simulink model "MMC_SwitchingModel_20250511"  (R2024b)
settings: Solver=VariableStepAuto  StartTime=0.0  StopTime=0.35  RelTol=1e-3
values from neighbouring files (symbols this model uses):
  Ceq = 3e-3    (= 0.003)    [param_allsim_20250429.m]
  f0 = 50    [param_allsim_20250429.m]
  Fc = 1e3    (= 1000)    [param_allsim_20250429.m]
  L_ac = 100e-6    (= 0.0001)    [param_allsim_20250429.m]
  L_arm = 1e-3    (= 0.001)    [param_allsim_20250429.m]
  m_Delta_0 = m_Delta_0_n    (= 0)    [param_allsim_20250429.m]
  m_Delta_d = M_Delta*sin(Phi_Delta)    [param_allsim_20250429.m]
  m_Delta_q = -M_Delta*cos(Phi_Delta)    [param_allsim_20250429.m]
  m_Sigma_0 = m_Sigma_0_n    (= 1)    [param_allsim_20250429.m]
  m_Sigma_d = M_Sigma*sin(Phi_Sigma)    [param_allsim_20250429.m]
  m_Sigma_q = -M_Sigma*cos(Phi_Sigma)    [param_allsim_20250429.m]
  N = 6    [param_allsim_20250429.m]
  R_ac = 1    [param_allsim_20250429.m]
  R_arm = 1e-2    (= 0.01)    [param_allsim_20250429.m]
  VDC = 800    [param_allsim_20250429.m]
undefined symbols (not defined in the file or in its folder): C_SM
libraries: spsVoltageMeasurementLib x11, spsCurrentMeasurementLib x8, spsSeriesRLCBranchLib x6, spsHalfBridgeMMCLib x6, spsPWMGeneratorMultilevelLib x6, spsabctodq0Lib x6, spsDCVoltageSourceLib x2, spsdq0toabcLib x2, spsGroundLib x1, spsThreePhaseSeriesRLCBranchLib x1, spsMeanLib x1, spspowerguiLib x1
(part 1 of 2)
settings Model: Creator=ana  LastModifiedBy=ana

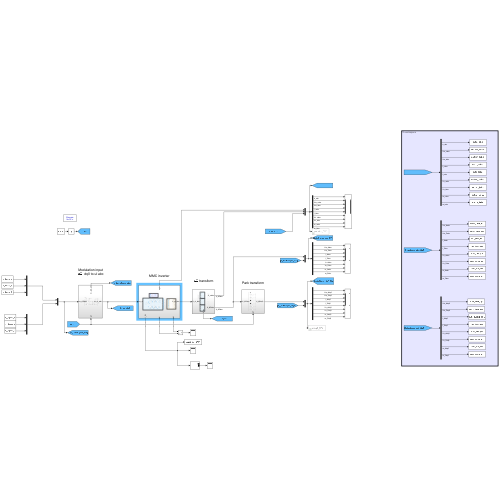
[thumbnail: Simulink's stored preview of the top-level diagram]
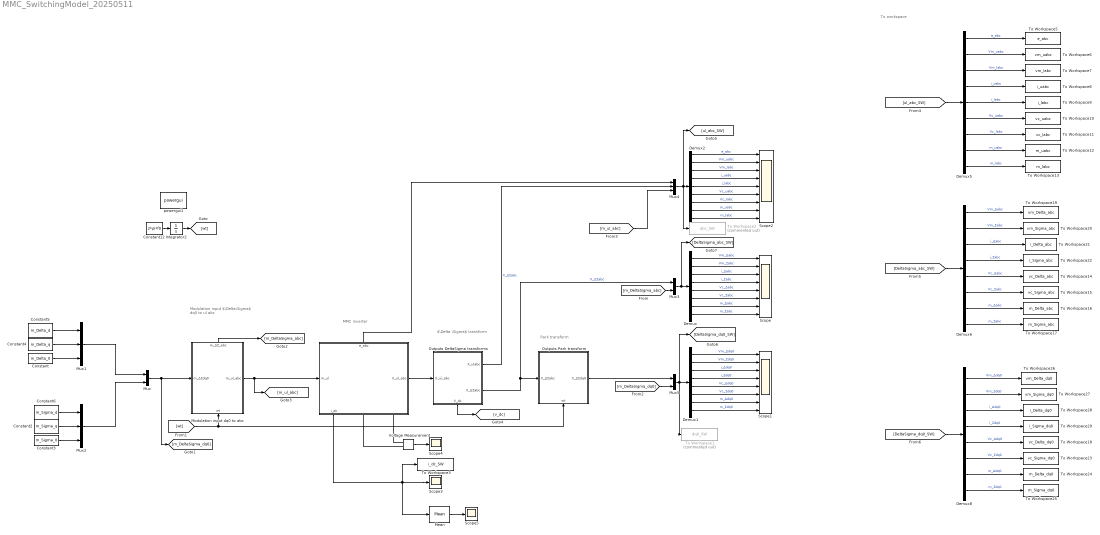
== system MMC_SwitchingModel_20250511 ==
  note: Modulation input
      | $\Delta\Sigma$ dq0 to ul abc
  note: MMC inverter
  note: $\Delta \Sigma$ transform
  note: Park transform
  note: To workspace
  " " : Subsystem
      settings: PortSchema="{\"entries\":[{\"content\":{\"sides\":[{\"content\":{\"connectorIds\":[\"In1\"]},\"type\":\"ConnectorPlacement.EquallySpacedRectSide\",\"uuid\":\"1684c177-0f69-459b-8ce9-190a6cc7c2f7\"},{\"content\":{\"connectorIds\":[\"Out1\"],\"side\":\"RIGHT\"},\"type\":\"ConnectorPlacement.EquallySpacedRectSide\",\"uuid\":\"0bff5431-30f2-45f3-9612-3e8ee114177b\"},{\"content\":{\"connectorIds\":[\"Out3\"],\"side\":\"TOP\"},\"type\":\"ConnectorPlacement.EquallySpacedRectSide\",\"uuid\":\"5880dbee-f5bf-4d11-b41f-6e883d19a036\"},{\"content\":{\"connectorIds\":[\"Out2\",\"RConn1\",\"RConn2\"],\"side\":\"BOTTOM\"},\"type\":\"ConnectorPlacement.EquallySpacedRectSide\",\"uuid\":\"e7f28e42-6c15-4753-aad9-7fd8153dbb2b\"}]},\"type\":\"ConnectorPlacement.EquallySpacedConnector\",\"uuid\":\"d5dc9c97-4c49-4fa9-8e0e-631ade92c721\"}],\"packageUris\":[\"http://schema.mathworks.com/mf0/Connector/R2020b\"],\"version\":\"1.0\"}"
  Constant : Constant  Value=m_Delta_0
  Constant12 : Constant  Value=2*pi*f0
  Constant2 : Constant  Value=m_Sigma_q
  Constant3 : Constant  Value=m_Sigma_0
  Constant4 : Constant  Value=m_Delta_q
  Constant5 : Constant  Value=m_Delta_d
  Constant6 : Constant  Value=m_Sigma_d  VectorParams1D=off
  Demux{,1,6,8} (4 alike) : Demux  Outputs=8
  Demux2 : Demux  Outputs=9
  Demux5 : Demux  Outputs=9
  Integrator2 : Integrator
  Mean : spsMeanLib/Mean  Freq=500  Vinit=0  Ts=0
  Modulation input dq0 to abc : Subsystem
      settings: PortSchema="{\"entries\":[{\"content\":{\"sides\":[{\"content\":{\"connectorIds\":[\"Out2\"]},\"type\":\"ConnectorPlacement.EquallySpacedRectSide\",\"uuid\":\"c93fa5b4-0f06-4bab-a3ea-c283951bfaa2\"},{\"content\":{\"connectorIds\":[\"In2\"],\"side\":\"RIGHT\"},\"type\":\"ConnectorPlacement.EquallySpacedRectSide\",\"uuid\":\"754fc415-ee26-4c64-88d9-9fe4c190d1ce\"},{\"content\":{\"connectorIds\":[\"Out1\"],\"side\":\"TOP\"},\"type\":\"ConnectorPlacement.EquallySpacedRectSide\",\"uuid\":\"5a2ac060-a673-4c08-b077-b80c57d082e2\"},{\"content\":{\"connectorIds\":[\"In1\"],\"side\":\"BOTTOM\"},\"type\":\"ConnectorPlacement.EquallySpacedRectSide\",\"uuid\":\"ce66d6e2-1782-404f-a52c-1b3df510631d\"}]},\"type\":\"ConnectorPlacement.EquallySpacedConnector\",\"uuid\":\"907f6fc0-1e89-4b6d-bca9-d0cf84d5397d\"}],\"packageUris\":[\"http://schema.mathworks.com/mf0/Connector/R2020b\"],\"version\":\"1.0\"}"
  Mux : Mux  Inputs=2
  Mux1 : Mux  Inputs=3
  Mux2 : Mux  Inputs=3
  Mux3 : Mux  Inputs=2
  Mux4 : Mux  Inputs=3
  Mux5 : Mux  Inputs=2
  Outputs DeltaSigma transforms : Subsystem
      settings: PortSchema="{\"entries\":[{\"content\":{\"sides\":[{\"content\":{\"connectorIds\":[\"Out2\",\"Out3\"]},\"type\":\"ConnectorPlacement.EquallySpacedRectSide\",\"uuid\":\"c93fa5b4-0f06-4bab-a3ea-c283951bfaa2\"},{\"content\":{\"connectorIds\":[\"In1\"],\"side\":\"RIGHT\"},\"type\":\"ConnectorPlacement.EquallySpacedRectSide\",\"uuid\":\"754fc415-ee26-4c64-88d9-9fe4c190d1ce\"},{\"content\":{\"side\":\"TOP\"},\"type\":\"ConnectorPlacement.EquallySpacedRectSide\",\"uuid\":\"5a2ac060-a673-4c08-b077-b80c57d082e2\"},{\"content\":{\"connectorIds\":[\"Out1\"],\"side\":\"BOTTOM\"},\"type\":\"ConnectorPlacement.EquallySpacedRectSide\",\"uuid\":\"ce66d6e2-1782-404f-a52c-1b3df510631d\"}]},\"type\":\"ConnectorPlacement.EquallySpacedConnector\",\"uuid\":\"907f6fc0-1e89-4b6d-bca9-d0cf84d5397d\"}],\"packageUris\":[\"http://schema.mathworks.com/mf0/Connector/R2020b\"],\"version\":\"1.0\"}"
  Outputs Park transform : Subsystem
      settings: PortSchema="{\"entries\":[{\"content\":{\"sides\":[{\"content\":{\"connectorIds\":[\"Out1\"]},\"type\":\"ConnectorPlacement.EquallySpacedRectSide\",\"uuid\":\"c93fa5b4-0f06-4bab-a3ea-c283951bfaa2\"},{\"content\":{\"connectorIds\":[\"In2\"],\"side\":\"RIGHT\"},\"type\":\"ConnectorPlacement.EquallySpacedRectSide\",\"uuid\":\"754fc415-ee26-4c64-88d9-9fe4c190d1ce\"},{\"content\":{\"side\":\"TOP\"},\"type\":\"ConnectorPlacement.EquallySpacedRectSide\",\"uuid\":\"5a2ac060-a673-4c08-b077-b80c57d082e2\"},{\"content\":{\"connectorIds\":[\"In1\"],\"side\":\"BOTTOM\"},\"type\":\"ConnectorPlacement.EquallySpacedRectSide\",\"uuid\":\"ce66d6e2-1782-404f-a52c-1b3df510631d\"}]},\"type\":\"ConnectorPlacement.EquallySpacedConnector\",\"uuid\":\"907f6fc0-1e89-4b6d-bca9-d0cf84d5397d\"}],\"packageUris\":[\"http://schema.mathworks.com/mf0/Connector/R2020b\"],\"version\":\"1.0\"}"
  Scope : Scope  NumInputPorts=8
  Scope1 : Scope  NumInputPorts=8
  Scope2 : Scope  NumInputPorts=9
  Scope3 : Scope
  Scope4 : Scope
  Scope5 : Scope
  To Workspace1 : ToWorkspace  Commented=on  VariableName=dq0_SW  SaveFormat=Structure With Time  SampleTime=-1
      settings: MaxDataPoints=round(10*2000*Fc/f0)
  To Workspace10 : ToWorkspace  VariableName=vc_uabc  SaveFormat=Structure With Time  SampleTime=-1
      settings: MaxDataPoints=10*200000
  To Workspace11 : ToWorkspace  VariableName=vc_labc  SaveFormat=Structure With Time  SampleTime=-1
      settings: MaxDataPoints=10*200000
  To Workspace12 : ToWorkspace  VariableName=m_uabc  SaveFormat=Structure With Time  SampleTime=-1
      settings: MaxDataPoints=10*200000
  To Workspace13 : ToWorkspace  VariableName=m_labc  SaveFormat=Structure With Time  SampleTime=-1
      settings: MaxDataPoints=10*200000
  To Workspace14 : ToWorkspace  VariableName=vc_Delta_abc  SaveFormat=Structure With Time  SampleTime=-1
      settings: MaxDataPoints=10*200000
  To Workspace15 : ToWorkspace  VariableName=vc_Sigma_abc  SaveFormat=Structure With Time  SampleTime=-1
      settings: MaxDataPoints=10*200000
  To Workspace16 : ToWorkspace  VariableName=m_Delta_abc  SaveFormat=Structure With Time  SampleTime=-1
      settings: MaxDataPoints=10*200000
  To Workspace17 : ToWorkspace  VariableName=m_Sigma_abc  SaveFormat=Structure With Time  SampleTime=-1
      settings: MaxDataPoints=10*200000
  To Workspace18 : ToWorkspace  VariableName=vc_Delta_dq0  SaveFormat=Structure With Time  SampleTime=-1
      settings: MaxDataPoints=10*200000
  To Workspace19 : ToWorkspace  VariableName=vm_Delta_abc  SaveFormat=Structure With Time  SampleTime=-1
      settings: MaxDataPoints=10*200000
  To Workspace2 : ToWorkspace  Commented=on  VariableName=abc_SW  SaveFormat=Structure With Time  SampleTime=-1
      settings: MaxDataPoints=round(10*2000*Fc/f0)
  To Workspace20 : ToWorkspace  VariableName=vm_Sigma_abc  SaveFormat=Structure With Time  SampleTime=-1
      settings: MaxDataPoints=10*200000
  To Workspace21 : ToWorkspace  VariableName=i_Delta_abc  SaveFormat=Structure With Time  SampleTime=-1
      settings: MaxDataPoints=10*200000
  To Workspace22 : ToWorkspace  VariableName=i_Sigma_abc  SaveFormat=Structure With Time  SampleTime=-1
      settings: MaxDataPoints=10*200000
  To Workspace23 : ToWorkspace  VariableName=vc_Sigma_dq0  SaveFormat=Structure With Time  SampleTime=-1
      settings: MaxDataPoints=10*200000
  To Workspace24 : ToWorkspace  VariableName=m_Delta_dq0  SaveFormat=Structure With Time  SampleTime=-1
      settings: MaxDataPoints=10*200000
  To Workspace25 : ToWorkspace  VariableName=m_Sigma_dq0  SaveFormat=Structure With Time  SampleTime=-1
      settings: MaxDataPoints=10*200000
  To Workspace26 : ToWorkspace  VariableName=vm_Delta_dq0  SaveFormat=Structure With Time  SampleTime=-1
      settings: MaxDataPoints=10*200000
  To Workspace27 : ToWorkspace  VariableName=vm_Sigma_dq0  SaveFormat=Structure With Time  SampleTime=-1
      settings: MaxDataPoints=10*200000
  To Workspace28 : ToWorkspace  VariableName=i_Delta_dq0  SaveFormat=Structure With Time  SampleTime=-1
      settings: MaxDataPoints=10*200000
  To Workspace29 : ToWorkspace  VariableName=i_Sigma_dq0  SaveFormat=Structure With Time  SampleTime=-1
      settings: MaxDataPoints=10*200000
  To Workspace3 : ToWorkspace  VariableName=i_dc_SW  SaveFormat=Structure With Time  SampleTime=-1
      settings: MaxDataPoints=round(10*2000*Fc/f0)
  To Workspace5 : ToWorkspace  VariableName=e_abc  SaveFormat=Structure With Time  SampleTime=-1
      settings: MaxDataPoints=10*200000
  To Workspace6 : ToWorkspace  VariableName=vm_uabc  SaveFormat=Structure With Time  SampleTime=-1
      settings: MaxDataPoints=10*200000
  To Workspace7 : ToWorkspace  VariableName=vm_labc  SaveFormat=Structure With Time  SampleTime=-1
      settings: MaxDataPoints=10*200000
  To Workspace8 : ToWorkspace  VariableName=i_uabc  SaveFormat=Structure With Time  SampleTime=-1
      settings: MaxDataPoints=10*200000
  To Workspace9 : ToWorkspace  VariableName=i_labc  SaveFormat=Structure With Time  SampleTime=-1
      settings: MaxDataPoints=10*200000
  Voltage Measurement : spsVoltageMeasurementLib/Voltage Measurement  PhasorSimulation=off  OutputType=Complex  PSBequivalent=0
  powergui1 : spspowerguiLib/powergui  Priority=1  SimulationMode=Discrete  SampleTime=1/(2000*Fc)  frequency=60  Iterations=50  frequencyindice=0  Pbase=100e6  ErrMax=1e-4  UnitsV=V  UnitsW=W  buscounter=0  FunctionMessages=off  echomessages=off  EnableUseOfTLC=off  CurrentSourceSwitches=off  DisableSnubberDevices=off  DisableRonSwitches=off  DisableVfSwitches=off  DisplayEquations=off  AutomaticDiscreteSolvers=off  SolverType=Backward Euler  Interpol=off  ExternalGateDelay=off  methode=off  Ts=0  x0status=blocks  SPID=off  SwTol=0  HookPort=off  NonlinearTolerance=1e-4  nMaxIteration=100  ContinueOnMaxIteration=off  RestoreLinks=warning  ResistiveCurrentMeasurement=off  Frange=[0:2:500]  Ylog=off  Xlog=on  ShowGrid=off  save=off  variable=ZData  structure=0  ZoomFFT=off  StartTime=0.0  cycles=1  DisplayStyle=1  fundamental=60  FreqAxis=off  MaxFrequency=1000  frequencyindicesteady=1  RmsSteady=1  display=off
  wires:
  Mux3/1 -> [DeltaSigma_abc_SW], Demux/1
  Mux/1 -> [m_DeltaSigma_dq0], Modulation input dq0 to abc/2(m_ΔΣdq0)
  " "/2(i_dc) -> To Workspace3/1, Scope3/1, Mean/1
  Demux1/7 -> Scope1/7  "m_Δdq0"
  Demux1/4 -> Scope1/4  "i_Σdq0"
  [m_ul_abc] -> Mux4/3
  [m_DeltaSigma_dq0] -> Mux5/2
  Demux1/3 -> Scope1/3  "i_Δdq0"
  Constant12/1 -> Integrator2/1
  " "/3(e_abc) -> Mux4/1
  Demux1/1 -> Scope1/1  "Vm_Δdq0"
  [wt] -> Outputs Park transform/1(wt), Modulation input dq0 to abc/1(wt)
  Modulation input dq0 to abc/2(m_ul_abc) -> [m_ul_abc], " "/1(m_ul)
  Demux1/2 -> Scope1/2  "Vm_Σdq0"
  Constant3/1 -> Mux2/3
  Outputs Park transform/1("X_ΔΣdq0 ") -> Mux5/1
  Demux/4 -> Scope/4  "i_Σabc"
  " "/1(X_ul_abc) -> Outputs DeltaSigma transforms/1(X_ul_abc)
  Outputs DeltaSigma transforms/2(X_ulabc) -> Mux4/2  "X_ΔΣabc"
  Mux2/1 -> Mux/2
  Mux1/1 -> Mux/1
  Mean/1 -> Scope5/1
  Constant2/1 -> Mux2/2
  Mux5/1 -> [DeltaSigma_dq0_SW], To Workspace1/1, Demux1/1
  Outputs DeltaSigma transforms/1(V_dc) -> [v_dc]
  Constant5/1 -> Mux1/1
  Demux1/5 -> Scope1/5  "Vc_Δdq0"
  Constant/1 -> Mux1/3
  Constant4/1 -> Mux1/2
  Constant6/1 -> Mux2/1
  Mux4/1 -> [ul_abc_SW], To Workspace2/1, Demux2/1
  Integrator2/1 -> [wt]
  Demux1/8 -> Scope1/8  "m_Σdq0"
  Demux1/6 -> Scope1/6  "Vc_Σdq0"
  Outputs DeltaSigma transforms/3(X_ΔΣabc) -> Mux3/1, Outputs Park transform/2("X_ΔΣabc ")  "X_ΔΣabc"
  Voltage Measurement/1 -> Scope4/1
  Modulation input dq0 to abc/1(m_ΔΣ_abc) -> [m_DeltaSigma_abc]
  [m_DeltaSigma_abc] -> Mux3/2
  Demux2/4 -> Scope2/4  "i_uabc"
  Demux2/9 -> Scope2/9  "m_labc"
  Demux2/2 -> Scope2/2  "Vm_uabc"
  Demux2/5 -> Scope2/5  "i_labc"
  Demux2/6 -> Scope2/6  "Vc_uabc"
  Demux2/7 -> Scope2/7  "Vc_labc"
  Demux2/8 -> Scope2/8  "m_uabc"
  Demux2/3 -> Scope2/3  "Vm_labc"
  Demux2/1 -> Scope2/1  "e_abc"
  Demux/1 -> Scope/1  "Vm_Δabc"
  Demux/6 -> Scope/6  "Vc_Σabc"
  Demux/3 -> Scope/3  "i_Δabc"
  Demux/2 -> Scope/2  "Vm_Σabc"
  Demux/8 -> Scope/8  "m_Σabc"
  Demux/7 -> Scope/7  "m_Δabc"
  Demux/5 -> Scope/5  "Vc_Δabc"
  Demux5/1 -> To Workspace5/1  "e_abc"
  Demux5/7 -> To Workspace11/1  "Vc_labc"
  Demux8/5 -> To Workspace18/1  "Vc_Δdq0"
  Demux6/2 -> To Workspace20/1  "Vm_Σabc"
  Demux8/4 -> To Workspace29/1  "i_Σdq0"
  Demux6/1 -> To Workspace19/1  "Vm_Δabc"
  Demux8/1 -> To Workspace26/1  "Vm_Δdq0"
  Demux6/8 -> To Workspace17/1  "m_Σabc"
  Demux8/3 -> To Workspace28/1  "i_Δdq0"
  Demux6/5 -> To Workspace14/1  "Vc_Δabc"
  Demux6/7 -> To Workspace16/1  "m_Δabc"
  Demux8/2 -> To Workspace27/1  "Vm_Σdq0"
  [ul_abc_SW] -> Demux5/1
  Demux8/7 -> To Workspace24/1  "m_Δdq0"
  Demux6/6 -> To Workspace15/1  "Vc_Σabc"
  Demux8/8 -> To Workspace25/1  "m_Σdq0"
  Demux6/4 -> To Workspace22/1  "i_Σabc"
  Demux5/5 -> To Workspace9/1  "i_labc"
  Demux6/3 -> To Workspace21/1  "i_Δabc"
  Demux5/2 -> To Workspace6/1  "Vm_uabc"
  [DeltaSigma_dq0_SW] -> Demux8/1
  [DeltaSigma_abc_SW] -> Demux6/1
  Demux5/3 -> To Workspace7/1  "Vm_labc"
  Demux5/9 -> To Workspace13/1  "m_labc"
  Demux5/4 -> To Workspace8/1  "i_uabc"
  Demux8/6 -> To Workspace23/1  "Vc_Σdq0"
  Demux5/6 -> To Workspace10/1  "Vc_uabc"
  Demux5/8 -> To Workspace12/1  "m_uabc"
  connections:
  Voltage Measurement/LConn1 -- " "/RConn1
  Voltage Measurement/LConn2 -- " "/RConn2

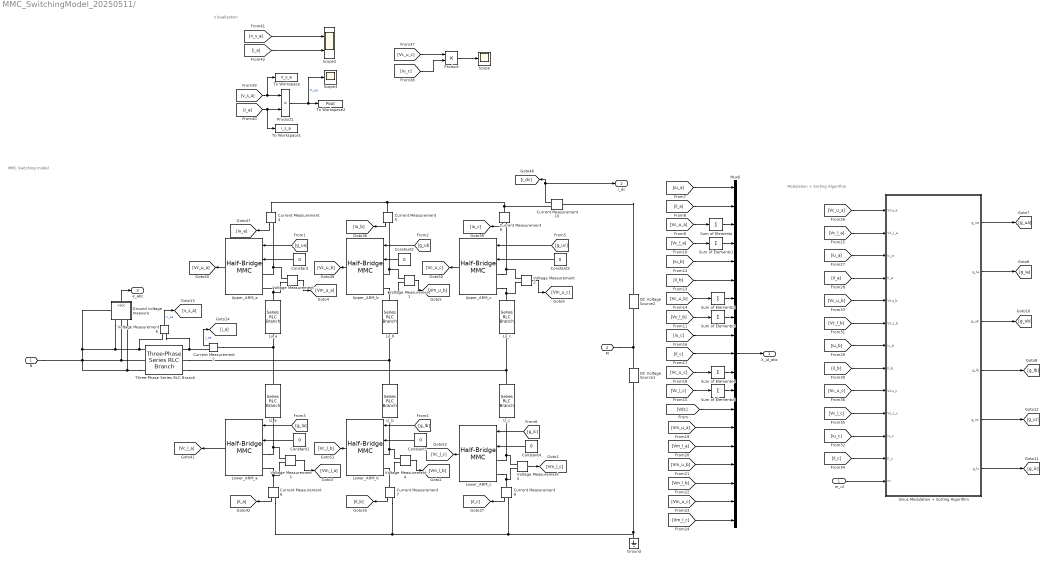
== system MMC_SwitchingModel_20250511/  ==
  note: Visualisation
  note: Modulation + Sorting Algorithm
  note: MMC Switching model
  m_ul : Inport
  Constant{,1..5} (6 alike) : Constant  Value=0
  Current Measurement{2,4..10} (8 alike) : spsCurrentMeasurementLib/Current Measurement  PhasorSimulation=off  OutputType=Complex  PSBequivalent=0
  DC Voltage Source1 : spsDCVoltageSourceLib/DC Voltage Source  Amplitude=VDC/2  Measurements=None
  DC Voltage Source2 : spsDCVoltageSourceLib/DC Voltage Source  Amplitude=VDC/2  Measurements=None
  Ground : spsGroundLib/Ground  LConnTagsString=a
  Ground voltage measure : Subsystem
      settings: PortSchema="{\"entries\":[{\"content\":{\"sides\":[{\"content\":{\"connectorIds\":[\"LConn1\",\"LConn2\",\"LConn3\"]},\"type\":\"ConnectorPlacement.EquallySpacedRectSide\",\"uuid\":\"2d863409-4ac8-4d89-98a2-a138b93b50bd\"},{\"content\":{\"connectorIds\":[\"Out1\"],\"side\":\"RIGHT\"},\"type\":\"ConnectorPlacement.EquallySpacedRectSide\",\"uuid\":\"6b7ceb28-dc80-4bb1-976d-3b9256003f0c\"},{\"content\":{\"connectorIds\":[\"LConn4\"],\"side\":\"TOP\"},\"type\":\"ConnectorPlacement.EquallySpacedRectSide\",\"uuid\":\"b87507a9-fcb6-4c8d-9886-4d479b5c7103\"}]},\"type\":\"ConnectorPlacement.EquallySpacedConnector\",\"uuid\":\"10f317e5-ccdd-49a1-b1ed-441de86b3420\"}],\"packageUris\":[\"http://schema.mathworks.com/mf0/Connector/R2020b\"],\"version\":\"1.0\"}"
  Ll_a : spsSeriesRLCBranchLib/Series RLC Branch  LConnTagsString=__new0  RConnTagsString=__new0  BranchType=RL  Resistance=R_arm  Inductance=L_arm  SetiL0=off  InitialCurrent=0  Capacitance=C_SM  Setx0=off  InitialVoltage=0  Measurements=None
  Ll_b : spsSeriesRLCBranchLib/Series RLC Branch  LConnTagsString=__new0  RConnTagsString=__new0  BranchType=RL  Resistance=R_arm  Inductance=L_arm  SetiL0=off  InitialCurrent=0  Capacitance=C_SM  Setx0=off  InitialVoltage=0  Measurements=None
  Ll_c : spsSeriesRLCBranchLib/Series RLC Branch  LConnTagsString=__new0  RConnTagsString=__new0  BranchType=RL  Resistance=R_arm  Inductance=L_arm  SetiL0=off  InitialCurrent=0  Capacitance=C_SM  Setx0=off  InitialVoltage=0  Measurements=None
  Lower_ARM_a : spsHalfBridgeMMCLib/Half-Bridge MMC  ModelType=Switching devices  n=N  C=Ceq*N  Vc_Initial=VDC/N  Ron=1e-4  Rs=1e6  Cs=inf  Ron_Diode=1e-3  Rs_Diode=1e6  Cs_Diode=inf  Vf_Diode=1e-3  Rs_CurrentSource=inf  Ts=10e-6
  Lower_ARM_b : spsHalfBridgeMMCLib/Half-Bridge MMC  ModelType=Switching devices  n=N  C=Ceq*N  Vc_Initial=VDC/N  Ron=1e-4  Rs=1e6  Cs=inf  Ron_Diode=1e-3  Rs_Diode=1e6  Cs_Diode=inf  Vf_Diode=1e-3  Rs_CurrentSource=inf  Ts=10e-6
  Lower_ARM_c : spsHalfBridgeMMCLib/Half-Bridge MMC  ModelType=Switching devices  n=N  C=Ceq*N  Vc_Initial=VDC/N  Ron=1e-4  Rs=1e6  Cs=inf  Ron_Diode=1e-3  Rs_Diode=1e6  Cs_Diode=inf  Vf_Diode=1e-3  Rs_CurrentSource=inf  Ts=10e-6
  Lu_a : spsSeriesRLCBranchLib/Series RLC Branch  LConnTagsString=__new0  RConnTagsString=__new0  BranchType=RL  Resistance=R_arm  Inductance=L_arm  SetiL0=off  InitialCurrent=0  Capacitance=C_SM  Setx0=off  InitialVoltage=0  Measurements=Branch voltage and current
  Lu_b : spsSeriesRLCBranchLib/Series RLC Branch  LConnTagsString=__new0  RConnTagsString=__new0  BranchType=RL  Resistance=R_arm  Inductance=L_arm  SetiL0=off  InitialCurrent=0  Capacitance=C_SM  Setx0=off  InitialVoltage=0  Measurements=Branch voltage and current
  Lu_c : spsSeriesRLCBranchLib/Series RLC Branch  LConnTagsString=__new0  RConnTagsString=__new0  BranchType=RL  Resistance=R_arm  Inductance=L_arm  SetiL0=off  InitialCurrent=0  Capacitance=C_SM  Setx0=off  InitialVoltage=0  Measurements=Branch voltage and current
  Mux6 : Mux  Inputs=19
  Product : Product
  Product1 : Product
  Scope : Scope
  Scope2 : Scope  NumInputPorts=2
  Scope3 : Scope
  Sinus Modulation + Sorting Algorithm : Subsystem
  Sum of Elements{,1..5} (6 alike) : Sum  Inputs=+
  Three-Phase Series RLC Branch : spsThreePhaseSeriesRLCBranchLib/Three-Phase Series RLC Branch  LConnTagsString=A|B|C  RConnTagsString=A|B|C  BranchType=RL  Resistance=R_ac  Inductance=L_ac  Capacitance=1e-6  Measurements=None
  To Workspace : ToWorkspace  VariableName=v_s_a  SaveFormat=Structure With Time  SampleTime=-1
  To Workspace1 : ToWorkspace  VariableName=i_s_a  SaveFormat=Structure With Time  SampleTime=-1
  To Workspace2 : ToWorkspace  VariableName=Pout  SaveFormat=Structure With Time  SampleTime=-1
  Upper_ARM_a : spsHalfBridgeMMCLib/Half-Bridge MMC  ModelType=Switching devices  n=N  C=Ceq*N  Vc_Initial=VDC/N  Ron=1e-4  Rs=1e6  Cs=inf  Ron_Diode=1e-3  Rs_Diode=1e6  Cs_Diode=inf  Vf_Diode=1e-3  Rs_CurrentSource=inf  Ts=10e-6
  Upper_ARM_b : spsHalfBridgeMMCLib/Half-Bridge MMC  ModelType=Switching devices  n=N  C=Ceq*N  Vc_Initial=VDC/N  Ron=1e-4  Rs=1e6  Cs=inf  Ron_Diode=1e-3  Rs_Diode=1e6  Cs_Diode=inf  Vf_Diode=1e-3  Rs_CurrentSource=inf  Ts=10e-6
  Upper_ARM_c : spsHalfBridgeMMCLib/Half-Bridge MMC  ModelType=Switching devices  n=N  C=Ceq*N  Vc_Initial=VDC/N  Ron=1e-4  Rs=1e6  Cs=inf  Ron_Diode=1e-3  Rs_Diode=1e6  Cs_Diode=inf  Vf_Diode=1e-3  Rs_CurrentSource=inf  Ts=10e-6
  Voltage Measurement{,1..6} (7 alike) : spsVoltageMeasurementLib/Voltage Measurement  PhasorSimulation=off  OutputType=Complex  PSBequivalent=0
  N : PMIOPort  Side=Right
  M : PMIOPort  Port=2  Side=Right
  X_ul_abc : Outport
  i_dc : Outport  Port=2
  e_abc : Outport  Port=3
  wires:
  [iu_a] -> Mux6/1
  [il_a] -> Mux6/2
  [Vc_u_a] -> Sum of Elements/1
  [Vc_l_a] -> Sum of Elements1/1
  [iu_b] -> Mux6/5
  [il_b] -> Mux6/6
  [Vc_u_b] -> Sum of Elements2/1
  [Vc_l_b] -> Sum of Elements3/1
  [iu_c] -> Mux6/9
  [il_c] -> Mux6/10
  [Vc_u_c] -> Sum of Elements4/1
  [Vc_l_c] -> Sum of Elements5/1
  Mux6/1 -> X_ul_abc/1
  [Vdc] -> Mux6/13
  [Vm_u_a] -> Mux6/14
  [Vm_l_a] -> Mux6/15
  [Vm_u_b] -> Mux6/16
  [Vm_l_b] -> Mux6/17
  [Vm_u_c] -> Mux6/18
  [Vm_l_c] -> Mux6/19
  Lower_ARM_b/1 -> [Vc_l_b]
  [g_lc] -> Lower_ARM_c/1
  Current Measurement5/1 -> [iu_b]
  Current Measurement6/1 -> [il_a]
  Constant2/1 -> Upper_ARM_b/2
  Current Measurement8/1 -> [iu_c]
  Upper_ARM_b/1 -> [Vc_u_b]
  [g_uc] -> Upper_ARM_c/1
  Constant3/1 -> Upper_ARM_c/2
  Lower_ARM_c/1 -> [Vc_l_c]
  [g_ub] -> Upper_ARM_b/1
  Current Measurement7/1 -> [il_b]
  Constant4/1 -> Lower_ARM_c/2
  [g_ua] -> Upper_ARM_a/1
  Constant/1 -> Upper_ARM_a/2
  Current Measurement4/1 -> [iu_a]
  Current Measurement9/1 -> [il_c]
  [g_lb] -> Lower_ARM_b/1
  Constant5/1 -> Lower_ARM_b/2
  [g_la] -> Lower_ARM_a/1
  Lower_ARM_a/1 -> [Vc_l_a]
  Constant1/1 -> Lower_ARM_a/2
  Upper_ARM_a/1 -> [Vc_u_a]
  Sinus Modulation + Sorting Algorithm/3(g_ub) -> [g_ub]
  Sinus Modulation + Sorting Algorithm/2(g_la) -> [g_la]
  Sinus Modulation + Sorting Algorithm/5(g_uc) -> [g_uc]
  Sinus Modulation + Sorting Algorithm/1(g_ua) -> [g_ua]
  Sinus Modulation + Sorting Algorithm/6(g_lc) -> [g_lc]
  [Vc_l_c] -> Sinus Modulation + Sorting Algorithm/10(Vc_l_c)
  Sinus Modulation + Sorting Algorithm/4(g_lb) -> [g_lb]
  [Vc_l_b] -> Sinus Modulation + Sorting Algorithm/6(Vc_l_b)
  [iu_a] -> Sinus Modulation + Sorting Algorithm/3(iu_a)
  [iu_c] -> Sinus Modulation + Sorting Algorithm/11(iu_c)
  [il_a] -> Sinus Modulation + Sorting Algorithm/4(Il_a)
  [Vc_u_b] -> Sinus Modulation + Sorting Algorithm/5(Vcu_b)
  [il_c] -> Sinus Modulation + Sorting Algorithm/12(Il_c)
  [Vc_u_a] -> Sinus Modulation + Sorting Algorithm/1(Vcu_a)
  [iu_b] -> Sinus Modulation + Sorting Algorithm/7(iu_b)
  [il_b] -> Sinus Modulation + Sorting Algorithm/8(Il_b)
  [Vc_l_a] -> Sinus Modulation + Sorting Algorithm/2(Vc_l_a)
  [Vc_u_c] -> Sinus Modulation + Sorting Algorithm/9(Vcu_c)
  m_ul/1 -> Sinus Modulation + Sorting Algorithm/13(m)
  Sum of Elements/1 -> Mux6/3
  Sum of Elements1/1 -> Mux6/4
  Sum of Elements2/1 -> Mux6/7
  Sum of Elements3/1 -> Mux6/8
  Sum of Elements4/1 -> Mux6/11
  Sum of Elements5/1 -> Mux6/12
  Upper_ARM_c/1 -> [Vc_u_c]
  Current Measurement10/1 -> i_dc/1, [i_dc]
  Ground voltage measure/1(vabc) -> e_abc/1
  [Vc_u_c] -> Product/1
  [iu_c] -> Product/2
  Product/1 -> Scope/1
  Voltage Measurement5/1 -> [Vm_l_c]
  Voltage Measurement4/1 -> [Vm_l_b]
  Voltage Measurement3/1 -> [Vm_l_a]
  Voltage Measurement/1 -> [Vm_u_a]
  Voltage Measurement1/1 -> [Vm_u_b]
  Voltage Measurement2/1 -> [Vm_u_c]
  Product1/1 -> Scope3/1, To Workspace2/1  "P_sa"
  Voltage Measurement6/1 -> [v_s_a]  "v_sa"
  Current Measurement2/1 -> [i_a]  "i_sa"
  [v_s_a] -> To Workspace/1, Product1/1
  [i_a] -> Product1/2, To Workspace1/1
  [v_s_a] -> Scope2/1
  [i_a] -> Scope2/2
  connections:
  Current Measurement6/RConn1 -- DC Voltage Source1/LConn1 -- Ground/LConn1 -- Current Measurement9/RConn1 -- Current Measurement7/RConn1
  DC Voltage Source1/RConn1 -- M/RConn1 -- DC Voltage Source2/LConn1
  Ll_c/LConn1 -- Lu_c/RConn1 -- Three-Phase Series RLC Branch/LConn3
  Ll_b/LConn1 -- Three-Phase Series RLC Branch/LConn2 -- Lu_b/RConn1
  Current Measurement5/LConn1 -- Current Measurement10/RConn1 -- Current Measurement8/LConn1 -- Current Measurement4/LConn1
  Ll_a/LConn1 -- Current Measurement2/LConn1 -- Lu_a/RConn1
  Current Measurement4/RConn1 -- Upper_ARM_a/LConn1 -- Voltage Measurement/LConn1
  Lower_ARM_b/LConn2 -- Voltage Measurement4/LConn2 -- Current Measurement7/LConn1
  Upper_ARM_b/LConn2 -- Voltage Measurement1/LConn2 -- Lu_b/LConn1
  Lower_ARM_a/LConn2 -- Voltage Measurement3/LConn2 -- Current Measurement6/LConn1
  Upper_ARM_c/LConn1 -- Voltage Measurement2/LConn1 -- Current Measurement8/RConn1
  Lower_ARM_b/LConn1 -- Voltage Measurement4/LConn1 -- Ll_b/RConn1
  Lower_ARM_c/LConn2 -- Voltage Measurement5/LConn2 -- Current Measurement9/LConn1
  Lower_ARM_a/LConn1 -- Voltage Measurement3/LConn1 -- Ll_a/RConn1
  Lu_a/LConn1 -- Upper_ARM_a/LConn2 -- Voltage Measurement/LConn2
  Upper_ARM_b/LConn1 -- Voltage Measurement1/LConn1 -- Current Measurement5/RConn1
  Lower_ARM_c/LConn1 -- Voltage Measurement5/LConn1 -- Ll_c/RConn1
  Upper_ARM_c/LConn2 -- Voltage Measurement2/LConn2 -- Lu_c/LConn1
  Three-Phase Series RLC Branch/RConn3 -- Three-Phase Series RLC Branch/RConn2 -- Ground voltage measure/LConn2 -- Voltage Measurement6/LConn2 -- Three-Phase Series RLC Branch/RConn1 -- Ground voltage measure/LConn1 -- Ground voltage measure/LConn4 -- N/RConn1 -- Ground voltage measure/LConn3
  DC Voltage Source2/RConn1 -- Current Measurement10/LConn1
  Voltage Measurement6/LConn1 -- Current Measurement2/RConn1 -- Three-Phase Series RLC Branch/LConn1

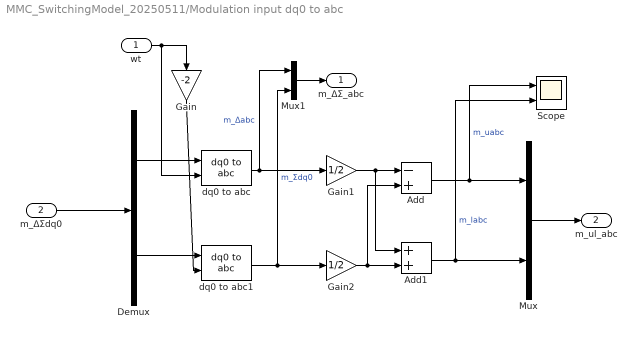
== system MMC_SwitchingModel_20250511/Modulation input dq0 to abc ==
  wt : Inport
  m_ΔΣdq0 : Inport  Port=2
  Add : Sum  Inputs=-+
  Add1 : Sum
  Demux : Demux  Outputs=2
  Gain : Gain  Gain=-2
  Gain1 : Gain  Gain=1/2
  Gain2 : Gain  Gain=1/2
  Mux : Mux  Inputs=2
  Mux1 : Mux  Inputs=2
  Scope : Scope  NumInputPorts=2
  dq0 to abc : spsdq0toabcLib/dq0 to abc  Alignment=Aligned with phase A axis
  dq0 to abc1 : spsdq0toabcLib/dq0 to abc  Alignment=Aligned with phase A axis
  m_ΔΣ_abc : Outport
  m_ul_abc : Outport  Port=2
  wires:
  m_ΔΣdq0/1 -> Demux/1
  wt/1 -> dq0 to abc/2, Gain/1
  Mux/1 -> m_ul_abc/1
  Demux/1 -> dq0 to abc/1
  Demux/2 -> dq0 to abc1/1
  Gain/1 -> dq0 to abc1/2
  dq0 to abc/1 -> Mux1/1, Gain1/1  "m_Δabc"
  dq0 to abc1/1 -> Mux1/2, Gain2/1  "m_Σdq0"
  Gain2/1 -> Add/2, Add1/2
  Gain1/1 -> Add1/1, Add/1
  Add/1 -> Scope/1, Mux/1  "m_uabc"
  Add1/1 -> Mux/2, Scope/2  "m_labc"
  Mux1/1 -> m_ΔΣ_abc/1

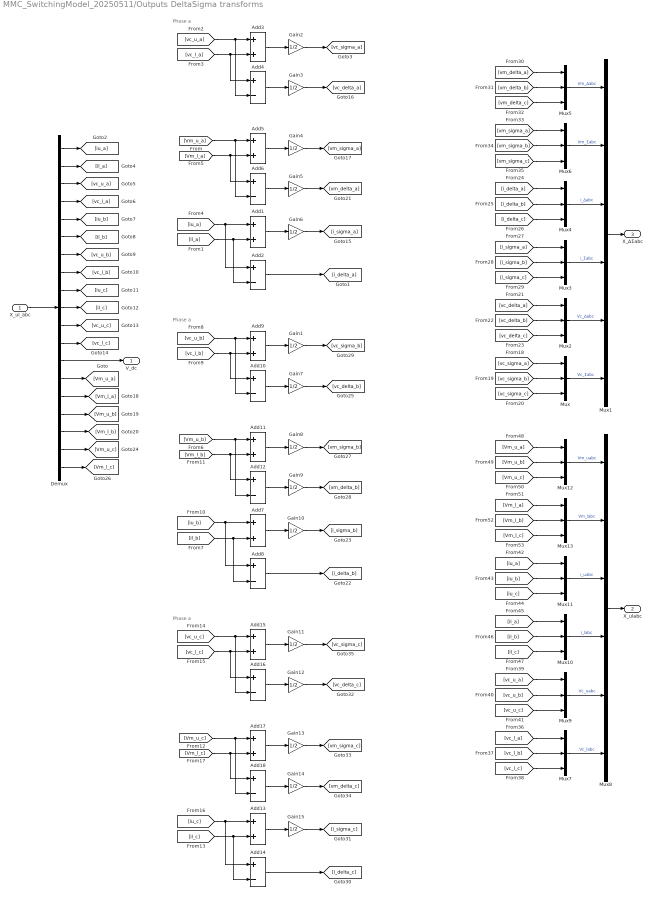
== system MMC_SwitchingModel_20250511/Outputs DeltaSigma transforms ==
  note: Phase a
  note: Phase a
  note: Phase a
  X_ul_abc : Inport
  Add{1,3,5,7,9,11,13,15,17} (9 alike) : Sum
  Add{2,4,6,8,10,12,14,16,18} (9 alike) : Sum  Inputs=+-
  Demux : Demux  Outputs=19
  Gain{1..15} (15 alike) : Gain  Gain=1/2
  Mux{,2..7,9..13} (12 alike) : Mux  Inputs=3
  Mux1 : Mux  Inputs=6
  Mux8 : Mux  Inputs=6
  V_dc : Outport
  X_ulabc : Outport  Port=2
  X_ΔΣabc : Outport  Port=3
  wires:
  X_ul_abc/1 -> Demux/1
  Demux/1 -> [iu_a]
  Demux/2 -> [il_a]
  Demux/3 -> [vc_u_a]
  Demux/4 -> [vc_l_a]
  Demux/5 -> [iu_b]
  Demux/6 -> [il_b]
  Demux/7 -> [vc_u_b]
  Demux/8 -> [vc_l_b]
  Demux/9 -> [iu_c]
  Demux/10 -> [il_c]
  Demux/11 -> [vc_u_c]
  Demux/12 -> [vc_l_c]
  Demux/13 -> V_dc/1
  [iu_a] -> Add2/1, Add1/1
  [vc_l_a] -> Add4/1, Add3/2
  [vc_u_a] -> Add4/2, Add3/1
  Gain2/1 -> [vc_sigma_a]
  Add1/1 -> Gain6/1
  Add3/1 -> Gain2/1
  [il_a] -> Add2/2, Add1/2
  Demux/14 -> [Vm_u_a]
  Demux/15 -> [Vm_l_a]
  Demux/16 -> [Vm_u_b]
  Demux/17 -> [Vm_l_b]
  Demux/18 -> [Vm_u_c]
  Demux/19 -> [Vm_l_c]
  Add4/1 -> Gain3/1
  Gain3/1 -> [vc_delta_a]
  Gain5/1 -> [vm_delta_a]
  Add6/1 -> Gain5/1
  Add5/1 -> Gain4/1
  [Vm_l_a] -> Add6/1, Add5/2
  Gain4/1 -> [vm_sigma_a]
  [Vm_u_a] -> Add6/2, Add5/1
  Add2/1 -> [i_delta_a]
  Gain6/1 -> [i_sigma_a]
  Gain8/1 -> [vm_sigma_b]
  Add11/1 -> Gain8/1
  Gain7/1 -> [vc_delta_b]
  Add10/1 -> Gain7/1
  [Vm_u_b] -> Add12/2, Add11/1
  Add9/1 -> Gain1/1
  [il_b] -> Add8/2, Add7/2
  Add7/1 -> Gain10/1
  Gain9/1 -> [vm_delta_b]
  [iu_b] -> Add8/1, Add7/1
  [vc_u_b] -> Add10/2, Add9/1
  Gain1/1 -> [vc_sigma_b]
  Add12/1 -> Gain9/1
  Add8/1 -> [i_delta_b]
  Gain10/1 -> [i_sigma_b]
  [Vm_l_b] -> Add12/1, Add11/2
  [vc_l_b] -> Add10/1, Add9/2
  Gain13/1 -> [vm_sigma_c]
  Add17/1 -> Gain13/1
  Gain12/1 -> [vc_delta_c]
  Add16/1 -> Gain12/1
  [Vm_u_c] -> Add18/2, Add17/1
  Add15/1 -> Gain11/1
  [il_c] -> Add14/2, Add13/2
  Add13/1 -> Gain15/1
  Gain14/1 -> [vm_delta_c]
  [iu_c] -> Add14/1, Add13/1
  [vc_u_c] -> Add16/2, Add15/1
  Gain11/1 -> [vc_sigma_c]
  Add18/1 -> Gain14/1
  Add14/1 -> [i_delta_c]
  Gain15/1 -> [i_sigma_c]
  [Vm_l_c] -> Add18/1, Add17/2
  [vc_l_c] -> Add16/1, Add15/2
  [vc_sigma_a] -> Mux/1
  [vc_sigma_b] -> Mux/2
  [vc_sigma_c] -> Mux/3
  [vc_delta_a] -> Mux2/1
  [vc_delta_b] -> Mux2/2
  [vc_delta_c] -> Mux2/3
  Mux2/1 -> Mux1/5  "Vc_Δabc"
  Mux/1 -> Mux1/6  "Vc_Σabc"
  Mux3/1 -> Mux1/4  "i_Σabc"
  [i_sigma_c] -> Mux3/3
  [i_sigma_b] -> Mux3/2
  [i_sigma_a] -> Mux3/1
  Mux4/1 -> Mux1/3  "i_Δabc"
  [i_delta_a] -> Mux4/1
  [i_delta_b] -> Mux4/2
  [i_delta_c] -> Mux4/3
  [vm_delta_b] -> Mux5/2
  [vm_delta_c] -> Mux5/3
  Mux5/1 -> Mux1/1  "Vm_Δabc"
  [vm_delta_a] -> Mux5/1
  [vm_sigma_a] -> Mux6/1
  [vm_sigma_c] -> Mux6/3
  [vm_sigma_b] -> Mux6/2
  Mux6/1 -> Mux1/2  "Vm_Σabc"
  Mux1/1 -> X_ΔΣabc/1
  [Vm_l_b] -> Mux13/2
  Mux9/1 -> Mux8/5  "Vc_uabc"
  [Vm_u_a] -> Mux12/1
  [vc_l_c] -> Mux7/3
  Mux10/1 -> Mux8/4  "i_labc"
  [il_b] -> Mux10/2
  [vc_u_c] -> Mux9/3
  [iu_b] -> Mux11/2
  [il_a] -> Mux10/1
  [Vm_l_a] -> Mux13/1
  [vc_l_a] -> Mux7/1
  [vc_l_b] -> Mux7/2
  [Vm_l_c] -> Mux13/3
  [iu_c] -> Mux11/3
  [vc_u_b] -> Mux9/2
  Mux11/1 -> Mux8/3  "i_uabc"
  [Vm_u_c] -> Mux12/3
  Mux13/1 -> Mux8/2  "Vm_labc"
  [il_c] -> Mux10/3
  [Vm_u_b] -> Mux12/2
  Mux7/1 -> Mux8/6  "Vc_labc"
  [iu_a] -> Mux11/1
  Mux8/1 -> X_ulabc/1
  Mux12/1 -> Mux8/1  "Vm_uabc"
  [vc_u_a] -> Mux9/1

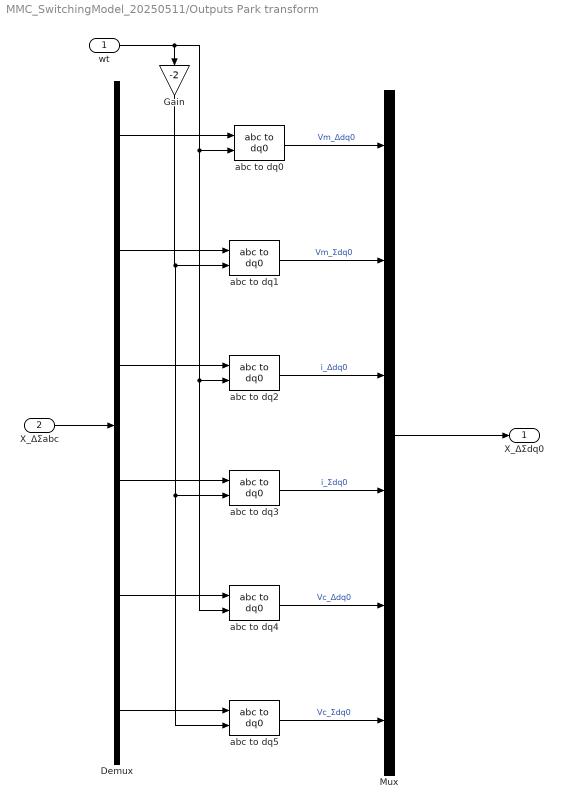
== system MMC_SwitchingModel_20250511/Outputs Park transform ==
  wt : Inport
  "X_ΔΣabc " : Inport  Port=2
  Demux : Demux  Outputs=6
  Gain : Gain  Gain=-2
  Mux : Mux  Inputs=6
  abc to dq{0..5} (6 alike) : spsabctodq0Lib/abc to dq0  Alignment=Aligned with phase A axis
  "X_ΔΣdq0 " : Outport
  wires:
  "X_ΔΣabc "/1 -> Demux/1
  Demux/1 -> abc to dq0/1
  wt/1 -> Gain/1, abc to dq4/2, abc to dq2/2, abc to dq0/2
  abc to dq0/1 -> Mux/1  "Vm_Δdq0"
  abc to dq1/1 -> Mux/2  "Vm_Σdq0"
  abc to dq2/1 -> Mux/3  "i_Δdq0"
  abc to dq3/1 -> Mux/4  "i_Σdq0"
  abc to dq4/1 -> Mux/5  "Vc_Δdq0"
  abc to dq5/1 -> Mux/6  "Vc_Σdq0"
  Gain/1 -> abc to dq1/2, abc to dq5/2, abc to dq3/2
  Demux/2 -> abc to dq1/1
  Demux/3 -> abc to dq2/1
  Demux/4 -> abc to dq3/1
  Demux/5 -> abc to dq4/1
  Demux/6 -> abc to dq5/1
  Mux/1 -> "X_ΔΣdq0 "/1

== system MMC_SwitchingModel_20250511/ /Ground voltage measure ==
  Mux : Mux  Inputs=3
  Voltage Measurement1 : spsVoltageMeasurementLib/Voltage Measurement  PhasorSimulation=off  OutputType=Complex  PSBequivalent=0
  Voltage Measurement2 : spsVoltageMeasurementLib/Voltage Measurement  PhasorSimulation=off  OutputType=Complex  PSBequivalent=0
  Voltage Measurement4 : spsVoltageMeasurementLib/Voltage Measurement  PhasorSimulation=off  OutputType=Complex  PSBequivalent=0
  a : PMIOPort  Side=Left
  b : PMIOPort  Port=2  Side=Left
  c : PMIOPort  Port=3  Side=Left
  N : PMIOPort  Port=4  Side=Left
  vabc : Outport
  wires:
  Voltage Measurement4/1 -> Mux/3
  Voltage Measurement2/1 -> Mux/2
  Mux/1 -> vabc/1
  Voltage Measurement1/1 -> Mux/1
  connections:
  Voltage Measurement2/LConn2 -- Voltage Measurement4/LConn2 -- N/RConn1 -- Voltage Measurement1/LConn2
  a/RConn1 -- Voltage Measurement1/LConn1
  b/RConn1 -- Voltage Measurement2/LConn1
  c/RConn1 -- Voltage Measurement4/LConn1

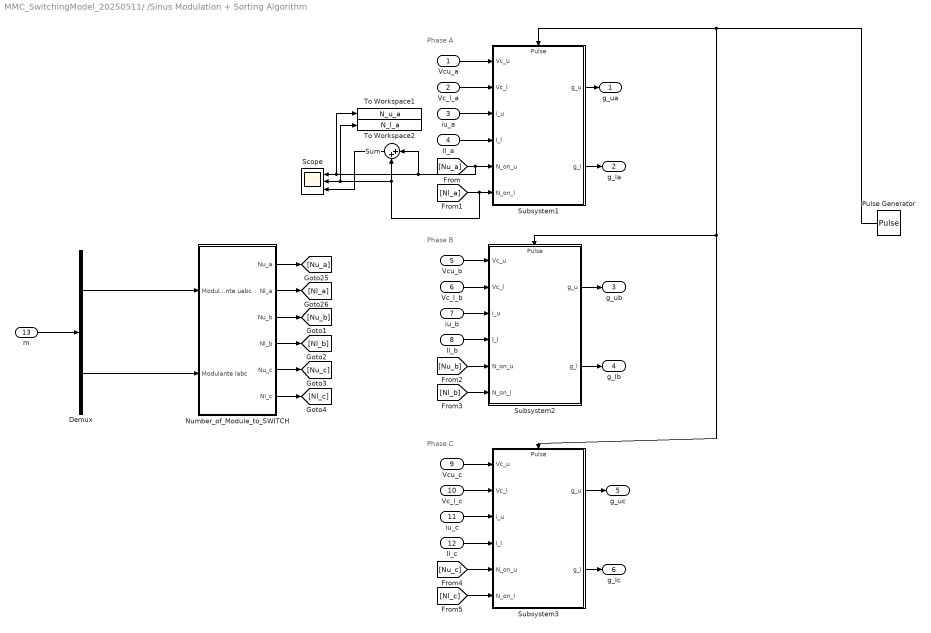
== system MMC_SwitchingModel_20250511/ /Sinus Modulation + Sorting Algorithm ==
  note: Phase A
  note: Phase B
  note: Phase C
  Vcu_a : Inport
  Vc_l_a : Inport  Port=2
  iu_a : Inport  Port=3
  Il_a : Inport  Port=4
  Vcu_b : Inport  Port=5
  Vc_l_b : Inport  Port=6
  iu_b : Inport  Port=7
  Il_b : Inport  Port=8
  Vcu_c : Inport  Port=9
  Vc_l_c : Inport  Port=10
  iu_c : Inport  Port=11
  Il_c : Inport  Port=12
  m : Inport  Port=13
  Demux : Demux  Outputs=2
  Number_of_Module_to_SWITCH : Subsystem
  Pulse Generator : DiscretePulseGenerator  PulseType=Time based  Period=1/(N*Fc)  SampleTime=1/(N*Fc)
  Scope : Scope  NumInputPorts=3
  Subsystem1 : Subsystem
      settings: PortSchema="{\"entries\":[{\"content\":{\"sides\":[{\"content\":{\"connectorIds\":[\"In1\",\"In2\",\"In3\",\"In4\",\"In5\",\"In6\"]},\"type\":\"ConnectorPlacement.EquallySpacedRectSide\",\"uuid\":\"edb50160-a239-40a6-972c-a715a6fbe13d\"},{\"content\":{\"connectorIds\":[\"Out1\",\"Out2\"],\"side\":\"RIGHT\"},\"type\":\"ConnectorPlacement.EquallySpacedRectSide\",\"uuid\":\"50795e67-0526-4c95-8fde-c2f33aa10269\"},{\"content\":{\"connectorIds\":[\"In7\"],\"side\":\"TOP\"},\"type\":\"ConnectorPlacement.EquallySpacedRectSide\",\"uuid\":\"4b9fa748-0c00-40fa-8ad9-db170ea8506d\"}]},\"type\":\"ConnectorPlacement.EquallySpacedConnector\",\"uuid\":\"80f12ca1-3964-4a1c-b648-ca12c0c72645\"}],\"packageUris\":[\"http://schema.mathworks.com/mf0/Connector/R2020b\"],\"version\":\"1.0\"}"
  Subsystem2 : Subsystem
      settings: PortSchema="{\"entries\":[{\"content\":{\"sides\":[{\"content\":{\"connectorIds\":[\"In1\",\"In2\",\"In3\",\"In4\",\"In5\",\"In6\"]},\"type\":\"ConnectorPlacement.EquallySpacedRectSide\",\"uuid\":\"edb50160-a239-40a6-972c-a715a6fbe13d\"},{\"content\":{\"connectorIds\":[\"Out1\",\"Out2\"],\"side\":\"RIGHT\"},\"type\":\"ConnectorPlacement.EquallySpacedRectSide\",\"uuid\":\"50795e67-0526-4c95-8fde-c2f33aa10269\"},{\"content\":{\"connectorIds\":[\"In7\"],\"side\":\"TOP\"},\"type\":\"ConnectorPlacement.EquallySpacedRectSide\",\"uuid\":\"4b9fa748-0c00-40fa-8ad9-db170ea8506d\"}]},\"type\":\"ConnectorPlacement.EquallySpacedConnector\",\"uuid\":\"80f12ca1-3964-4a1c-b648-ca12c0c72645\"}],\"packageUris\":[\"http://schema.mathworks.com/mf0/Connector/R2020b\"],\"version\":\"1.0\"}"
  Subsystem3 : Subsystem
      settings: PortSchema="{\"entries\":[{\"content\":{\"sides\":[{\"content\":{\"connectorIds\":[\"In1\",\"In2\",\"In3\",\"In4\",\"In5\",\"In6\"]},\"type\":\"ConnectorPlacement.EquallySpacedRectSide\",\"uuid\":\"edb50160-a239-40a6-972c-a715a6fbe13d\"},{\"content\":{\"connectorIds\":[\"Out1\",\"Out2\"],\"side\":\"RIGHT\"},\"type\":\"ConnectorPlacement.EquallySpacedRectSide\",\"uuid\":\"50795e67-0526-4c95-8fde-c2f33aa10269\"},{\"content\":{\"connectorIds\":[\"In7\"],\"side\":\"TOP\"},\"type\":\"ConnectorPlacement.EquallySpacedRectSide\",\"uuid\":\"4b9fa748-0c00-40fa-8ad9-db170ea8506d\"}]},\"type\":\"ConnectorPlacement.EquallySpacedConnector\",\"uuid\":\"80f12ca1-3964-4a1c-b648-ca12c0c72645\"}],\"packageUris\":[\"http://schema.mathworks.com/mf0/Connector/R2020b\"],\"version\":\"1.0\"}"
  Sum : Sum  Inputs=|++
  To Workspace1 : ToWorkspace  VariableName=N_u_a  SaveFormat=Structure With Time  SampleTime=-1
  To Workspace2 : ToWorkspace  VariableName=N_l_a  SaveFormat=Structure With Time  SampleTime=-1
  g_ua : Outport
  g_la : Outport  Port=2
  g_ub : Outport  Port=3
  g_lb : Outport  Port=4
  g_uc : Outport  Port=5
  g_lc : Outport  Port=6
  wires:
  Subsystem1/1(g_u) -> g_ua/1
  Il_a/1 -> Subsystem1/4(I_l)
  Subsystem1/2(g_l) -> g_la/1
  Vcu_a/1 -> Subsystem1/1(Vc_u)
  Vc_l_a/1 -> Subsystem1/2(Vc_l)
  iu_a/1 -> Subsystem1/3(i_u)
  [Nu_a] -> Sum/1, To Workspace1/1, Scope/1, Subsystem1/5(N_on_u)
  [Nl_a] -> Scope/2, To Workspace2/1, Sum/2, Subsystem1/6(N_on_l)
  iu_b/1 -> Subsystem2/3(i_u)
  Il_b/1 -> Subsystem2/4(I_l)
  Vcu_b/1 -> Subsystem2/1(Vc_u)
  Vc_l_b/1 -> Subsystem2/2(Vc_l)
  [Nu_b] -> Subsystem2/5(N_on_u)
  Subsystem2/2(g_l) -> g_lb/1
  [Nl_b] -> Subsystem2/6(N_on_l)
  Subsystem2/1(g_u) -> g_ub/1
  iu_c/1 -> Subsystem3/3(i_u)
  Il_c/1 -> Subsystem3/4(I_l)
  Vcu_c/1 -> Subsystem3/1(Vc_u)
  Vc_l_c/1 -> Subsystem3/2(Vc_l)
  [Nu_c] -> Subsystem3/5(N_on_u)
  [Nl_c] -> Subsystem3/6(N_on_l)
  Number_of_Module_to_SWITCH/3(Nu_b) -> [Nu_b]
  Number_of_Module_to_SWITCH/2(Nl_a) -> [Nl_a]
  Number_of_Module_to_SWITCH/6(Nl_c) -> [Nl_c]
  Number_of_Module_to_SWITCH/5(Nu_c) -> [Nu_c]
  Number_of_Module_to_SWITCH/4(Nl_b) -> [Nl_b]
  Number_of_Module_to_SWITCH/1(Nu_a) -> [Nu_a]
  m/1 -> Demux/1
  Demux/1 -> Number_of_Module_to_SWITCH/1(Modulante uabc)
  Demux/2 -> Number_of_Module_to_SWITCH/2(Modulante labc)
  Subsystem3/1(g_u) -> g_uc/1
  Subsystem3/2(g_l) -> g_lc/1
  Pulse Generator/1 -> Subsystem3/7(Pulse), Subsystem2/7(Pulse), Subsystem1/7(Pulse)
  Sum/1 -> Scope/3

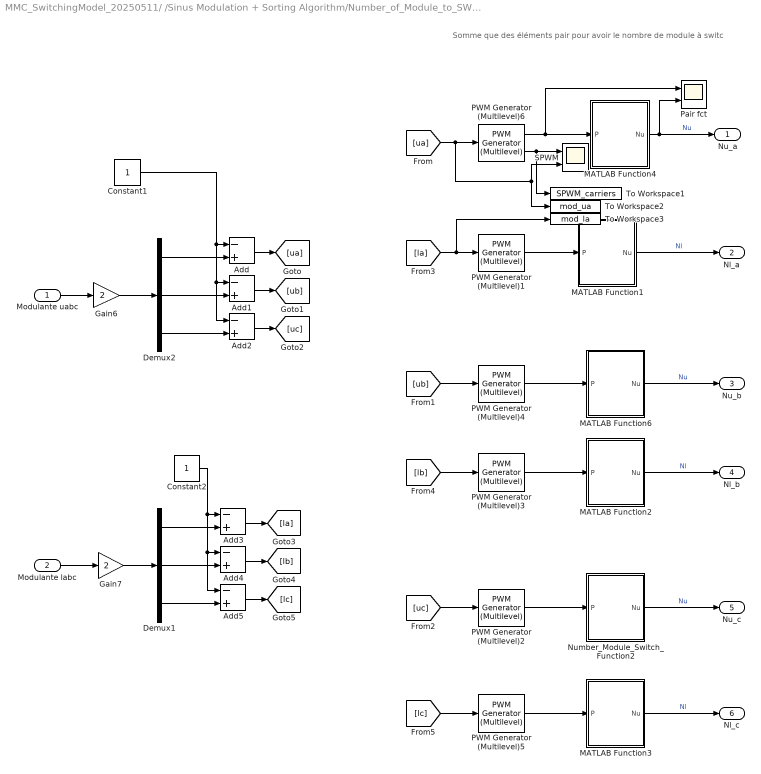
== system MMC_SwitchingModel_20250511/ /Sinus Modulation + Sorting Algorithm/Number_of_Module_to_SWITCH ==
  note: Somme que des éléments pair pour avoir le nombre de module à switc
  Modulante uabc : Inport
  Modulante labc : Inport  Port=2
  Add{,1..5} (6 alike) : Sum  Inputs=-+
  Constant1 : Constant
  Constant2 : Constant
  Demux1 : Demux  Outputs=3
  Demux2 : Demux  Outputs=3
  Gain6 : Gain  Gain=2
  Gain7 : Gain  Gain=2
  MATLAB Function1 : MATLAB Function  TreatAsAtomicUnit=on
  MATLAB Function2 : MATLAB Function  TreatAsAtomicUnit=on
  MATLAB Function3 : MATLAB Function  TreatAsAtomicUnit=on
  MATLAB Function4 : MATLAB Function  TreatAsAtomicUnit=on
  MATLAB Function6 : MATLAB Function  TreatAsAtomicUnit=on
  Number_Module_Switch_Function2 : MATLAB Function  TreatAsAtomicUnit=on
  PWM Generator (Multilevel){1..5} (5 alike) : spsPWMGeneratorMultilevelLib/PWM Generator (Multilevel)  BridgeType=Half-bridge  NumberOfBridges=N  Fc=Fc  Ts=0  ShowCarriersOutport=off
  PWM Generator (Multilevel)6 : spsPWMGeneratorMultilevelLib/PWM Generator (Multilevel)  BridgeType=Half-bridge  NumberOfBridges=N  Fc=Fc  Ts=0  ShowCarriersOutport=on
  Pair fct : Scope  NumInputPorts=2
  SPWM : Scope  NumInputPorts=2
  To Workspace1 : ToWorkspace  VariableName=SPWM_carriers  SaveFormat=Structure With Time  SampleTime=-1
  To Workspace2 : ToWorkspace  VariableName=mod_ua  SaveFormat=Structure With Time  SampleTime=-1
  To Workspace3 : ToWorkspace  VariableName=mod_la  SaveFormat=Structure With Time  SampleTime=-1
  Nu_a : Outport
  Nl_a : Outport  Port=2
  Nu_b : Outport  Port=3
  Nl_b : Outport  Port=4
  Nu_c : Outport  Port=5
  Nl_c : Outport  Port=6
  wires:
  Modulante uabc/1 -> Gain6/1
  PWM Generator (Multilevel)6/1 -> Pair fct/1, MATLAB Function4/1(P)
  [ua] -> To Workspace2/1, SPWM/2, PWM Generator (Multilevel)6/1
  MATLAB Function4/1(Nu) -> Pair fct/2, Nu_a/1  "Nu"
  PWM Generator (Multilevel)2/1 -> Number_Module_Switch_Function2/1(P)
  [ub] -> PWM Generator (Multilevel)4/1
  PWM Generator (Multilevel)4/1 -> MATLAB Function6/1(P)
  [uc] -> PWM Generator (Multilevel)2/1
  Modulante labc/1 -> Gain7/1
  MATLAB Function6/1(Nu) -> Nu_b/1  "Nu"
  Number_Module_Switch_Function2/1(Nu) -> Nu_c/1  "Nu"
  Demux2/1 -> Add/2
  Add/1 -> [ua]
  Demux2/2 -> Add1/2
  Add1/1 -> [ub]
  Demux2/3 -> Add2/2
  Add2/1 -> [uc]
  Constant1/1 -> Add2/1, Add1/1, Add/1
  Add5/1 -> [lc]
  Demux1/3 -> Add5/2
  Demux1/2 -> Add4/2
  Add4/1 -> [lb]
  Constant2/1 -> Add5/1, Add4/1, Add3/1
  Add3/1 -> [la]
  Demux1/1 -> Add3/2
  [la] -> To Workspace3/1, PWM Generator (Multilevel)1/1
  PWM Generator (Multilevel)1/1 -> MATLAB Function1/1(P)
  MATLAB Function1/1(Nu) -> Nl_a/1  "Nl"
  PWM Generator (Multilevel)3/1 -> MATLAB Function2/1(P)
  [lb] -> PWM Generator (Multilevel)3/1
  MATLAB Function2/1(Nu) -> Nl_b/1  "Nl"
  PWM Generator (Multilevel)5/1 -> MATLAB Function3/1(P)
  [lc] -> PWM Generator (Multilevel)5/1
  MATLAB Function3/1(Nu) -> Nl_c/1  "Nl"
  Gain6/1 -> Demux2/1
  Gain7/1 -> Demux1/1
  PWM Generator (Multilevel)6/2 -> To Workspace1/1, SPWM/1

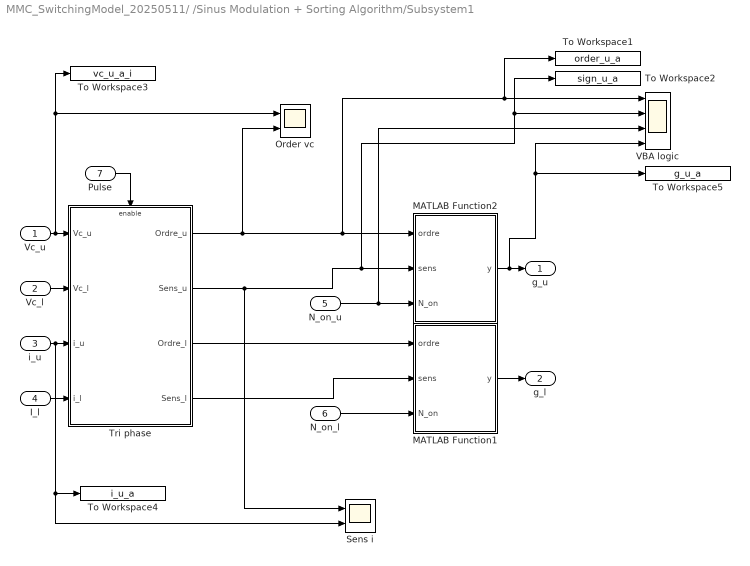
== system MMC_SwitchingModel_20250511/ /Sinus Modulation + Sorting Algorithm/Subsystem1 ==
  Vc_u : Inport
  Vc_l : Inport  Port=2
  i_u : Inport  Port=3
  I_l : Inport  Port=4
  N_on_u : Inport  Port=5
  N_on_l : Inport  Port=6
  Pulse : Inport  Port=7
  MATLAB Function1 : MATLAB Function  TreatAsAtomicUnit=on
  MATLAB Function2 : MATLAB Function  TreatAsAtomicUnit=on
  Order vc : Scope  NumInputPorts=2
  Sens i : Scope  NumInputPorts=2
  To Workspace1 : ToWorkspace  VariableName=order_u_a  SaveFormat=Structure With Time  SampleTime=-1
  To Workspace2 : ToWorkspace  VariableName=sign_u_a  SaveFormat=Structure With Time  SampleTime=-1
  To Workspace3 : ToWorkspace  VariableName=vc_u_a_i  SaveFormat=Structure With Time  SampleTime=-1
  To Workspace4 : ToWorkspace  VariableName=i_u_a  SaveFormat=Structure With Time  SampleTime=-1
  To Workspace5 : ToWorkspace  VariableName=g_u_a  SaveFormat=Structure With Time  SampleTime=-1
  Tri phase : Subsystem
  VBA logic : Scope  NumInputPorts=4
  g_u : Outport
  g_l : Outport  Port=2
  wires:
  Vc_u/1 -> To Workspace3/1, Order vc/1, Tri phase/1(Vc_u)
  Vc_l/1 -> Tri phase/2(Vc_l)
  Tri phase/1(Ordre_u) -> To Workspace1/1, VBA logic/1, MATLAB Function2/1(ordre), Order vc/2
  N_on_u/1 -> VBA logic/3, MATLAB Function2/3(N_on)
  i_u/1 -> To Workspace4/1, Sens i/2, Tri phase/3(i_u)
  Tri phase/2(Sens_u) -> Sens i/1, VBA logic/2, To Workspace2/1, MATLAB Function2/2(sens)
  Pulse/1 -> Tri phase/Enable
  I_l/1 -> Tri phase/4(i_l)
  Tri phase/3(Ordre_l) -> MATLAB Function1/1(ordre)
  N_on_l/1 -> MATLAB Function1/3(N_on)
  Tri phase/4(Sens_l) -> MATLAB Function1/2(sens)
  MATLAB Function1/1(y) -> g_l/1
  MATLAB Function2/1(y) -> To Workspace5/1, VBA logic/4, g_u/1

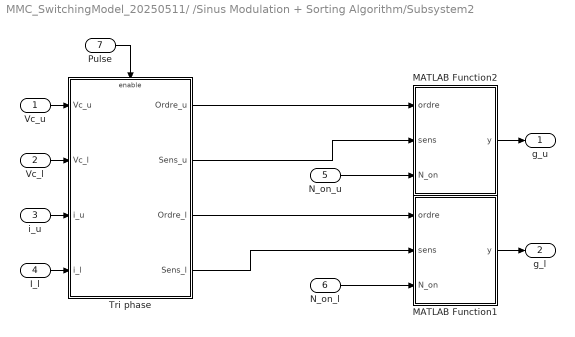
== system MMC_SwitchingModel_20250511/ /Sinus Modulation + Sorting Algorithm/Subsystem2 ==
  Vc_u : Inport
  Vc_l : Inport  Port=2
  i_u : Inport  Port=3
  I_l : Inport  Port=4
  N_on_u : Inport  Port=5
  N_on_l : Inport  Port=6
  Pulse : Inport  Port=7
  MATLAB Function1 : MATLAB Function  TreatAsAtomicUnit=on
  MATLAB Function2 : MATLAB Function  TreatAsAtomicUnit=on
  Tri phase : Subsystem
  g_u : Outport
  g_l : Outport  Port=2
  wires:
  Vc_u/1 -> Tri phase/1(Vc_u)
  Vc_l/1 -> Tri phase/2(Vc_l)
  Tri phase/1(Ordre_u) -> MATLAB Function2/1(ordre)
  N_on_u/1 -> MATLAB Function2/3(N_on)
  i_u/1 -> Tri phase/3(i_u)
  Tri phase/2(Sens_u) -> MATLAB Function2/2(sens)
  Pulse/1 -> Tri phase/Enable
  I_l/1 -> Tri phase/4(i_l)
  Tri phase/3(Ordre_l) -> MATLAB Function1/1(ordre)
  N_on_l/1 -> MATLAB Function1/3(N_on)
  Tri phase/4(Sens_l) -> MATLAB Function1/2(sens)
  MATLAB Function1/1(y) -> g_l/1
  MATLAB Function2/1(y) -> g_u/1

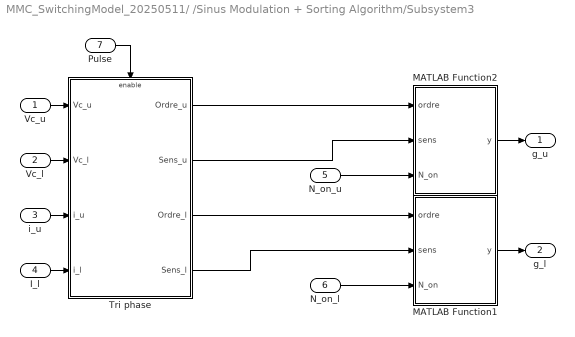
== system MMC_SwitchingModel_20250511/ /Sinus Modulation + Sorting Algorithm/Subsystem3 ==
  Vc_u : Inport
  Vc_l : Inport  Port=2
  i_u : Inport  Port=3
  I_l : Inport  Port=4
  N_on_u : Inport  Port=5
  N_on_l : Inport  Port=6
  Pulse : Inport  Port=7
  MATLAB Function1 : MATLAB Function  TreatAsAtomicUnit=on
  MATLAB Function2 : MATLAB Function  TreatAsAtomicUnit=on
  Tri phase : Subsystem
  g_u : Outport
  g_l : Outport  Port=2
  wires:
  Vc_u/1 -> Tri phase/1(Vc_u)
  Vc_l/1 -> Tri phase/2(Vc_l)
  Tri phase/1(Ordre_u) -> MATLAB Function2/1(ordre)
  N_on_u/1 -> MATLAB Function2/3(N_on)
  i_u/1 -> Tri phase/3(i_u)
  Tri phase/2(Sens_u) -> MATLAB Function2/2(sens)
  Pulse/1 -> Tri phase/Enable
  I_l/1 -> Tri phase/4(i_l)
  Tri phase/3(Ordre_l) -> MATLAB Function1/1(ordre)
  N_on_l/1 -> MATLAB Function1/3(N_on)
  Tri phase/4(Sens_l) -> MATLAB Function1/2(sens)
  MATLAB Function1/1(y) -> g_l/1
  MATLAB Function2/1(y) -> g_u/1

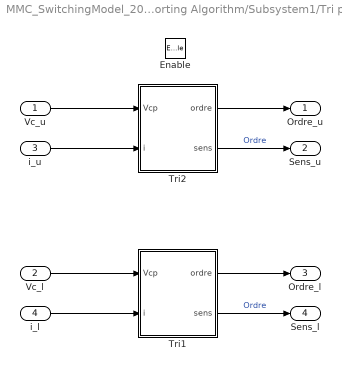
== system MMC_SwitchingModel_20250511/ /Sinus Modulation + Sorting Algorithm/Subsystem1/Tri phase ==
  Vc_u : Inport
  Vc_l : Inport  Port=2
  i_u : Inport  Port=3
  i_l : Inport  Port=4
  Enable : EnablePort
  Tri1 : MATLAB Function  TreatAsAtomicUnit=on
  Tri2 : MATLAB Function  TreatAsAtomicUnit=on
  Ordre_u : Outport
  Sens_u : Outport  Port=2
  Ordre_l : Outport  Port=3
  Sens_l : Outport  Port=4
  wires:
  Vc_u/1 -> Tri2/1(Vcp)
  i_u/1 -> Tri2/2(i)
  Vc_l/1 -> Tri1/1(Vcp)
  i_l/1 -> Tri1/2(i)
  Tri2/1(ordre) -> Ordre_u/1
  Tri2/2(sens) -> Sens_u/1  "Ordre"
  Tri1/2(sens) -> Sens_l/1  "Ordre"
  Tri1/1(ordre) -> Ordre_l/1

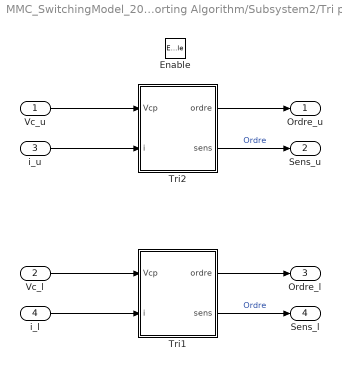
== system MMC_SwitchingModel_20250511/ /Sinus Modulation + Sorting Algorithm/Subsystem2/Tri phase ==
  Vc_u : Inport
  Vc_l : Inport  Port=2
  i_u : Inport  Port=3
  i_l : Inport  Port=4
  Enable : EnablePort
  Tri1 : MATLAB Function  TreatAsAtomicUnit=on
  Tri2 : MATLAB Function  TreatAsAtomicUnit=on
  Ordre_u : Outport
  Sens_u : Outport  Port=2
  Ordre_l : Outport  Port=3
  Sens_l : Outport  Port=4
  wires:
  Vc_u/1 -> Tri2/1(Vcp)
  i_u/1 -> Tri2/2(i)
  Vc_l/1 -> Tri1/1(Vcp)
  i_l/1 -> Tri1/2(i)
  Tri2/1(ordre) -> Ordre_u/1
  Tri2/2(sens) -> Sens_u/1  "Ordre"
  Tri1/2(sens) -> Sens_l/1  "Ordre"
  Tri1/1(ordre) -> Ordre_l/1

== system MMC_SwitchingModel_20250511/ /Sinus Modulation + Sorting Algorithm/Subsystem3/Tri phase ==
  Vc_u : Inport
  Vc_l : Inport  Port=2
  i_u : Inport  Port=3
  i_l : Inport  Port=4
  Enable : EnablePort
  Tri1 : MATLAB Function  TreatAsAtomicUnit=on
  Tri2 : MATLAB Function  TreatAsAtomicUnit=on
  Ordre_u : Outport
  Sens_u : Outport  Port=2
  Ordre_l : Outport  Port=3
  Sens_l : Outport  Port=4
  wires:
  Vc_u/1 -> Tri2/1(Vcp)
  i_u/1 -> Tri2/2(i)
  Vc_l/1 -> Tri1/1(Vcp)
  i_l/1 -> Tri1/2(i)
  Tri2/1(ordre) -> Ordre_u/1
  Tri2/2(sens) -> Sens_u/1  "Ordre"
  Tri1/2(sens) -> Sens_l/1  "Ordre"
  Tri1/1(ordre) -> Ordre_l/1

== matlab function MMC_SwitchingModel_20250511/ /Sinus Modulation + Sorting Algorithm/Subsystem2/MATLAB Function1 ==
  data: ordre input; y output; sens input; N_on input
function y = fcn(ordre,sens,N_on)

N_m = length(ordre);
Gp = zeros(1,2*N_m);
Ap0=ordre;

%% Sens positif (sens = 1)
if sens==1         % ON les condensateurs les moins chargés
    
    %K1 = 1 ; K2 = 0
    kp = 1:N_on;
    Gp(2*Ap0(kp))=0;
    Gp(2*Ap0(kp)-1)=1;
    
    %K1 = 0 ; K2 = 1
    kp = N_on+1:N_m;
    Gp(2*Ap0(kp))=1;
    Gp(2*Ap0(kp)-1)=0;

else            % ON les condensateurs les plus chargés
    
    %K1 = 1 ; K2 = 0
    kp = N_m:-1:N_m+1-N_on;
    Gp(2*Ap0(kp))=0;
    Gp(2*Ap0(kp)-1)=1;
    
    %K1 = 0 ; K2 = 1
    kp = N_m-N_on:-1:1;
    Gp(2*Ap0(kp))=1;
    Gp(2*Ap0(kp)-1)=0;
end
y=Gp;

== matlab function MMC_SwitchingModel_20250511/ /Sinus Modulation + Sorting Algorithm/Subsystem1/Tri phase/Tri1 ==
  data: ordre output; Vcp input; i input; sens output
function [ordre,sens] = fcn(Vcp, i)

[~, ordre] = sort(Vcp);

if i > 0 
    sens = 1;
else 
    sens = 0;
end

== matlab function MMC_SwitchingModel_20250511/ /Sinus Modulation + Sorting Algorithm/Subsystem1/MATLAB Function2 ==
  data: ordre input; y output; sens input; N_on input
function y = fcn(ordre,sens,N_on)

N_m = length(ordre);
Gp = zeros(1,2*N_m);
Ap0=ordre;

%% Sens positif (sens = 1)
if sens==1         % ON les condensateurs les moins chargés
    
    %K1 = 1 ; K2 = 0
    kp = 1:N_on;
    Gp(2*Ap0(kp))=0;
    Gp(2*Ap0(kp)-1)=1;
    
    %K1 = 0 ; K2 = 1
    kp = N_on+1:N_m;
    Gp(2*Ap0(kp))=1;
    Gp(2*Ap0(kp)-1)=0;

else            % ON les condensateurs les plus chargés
    
    %K1 = 1 ; K2 = 0
    kp = N_m:-1:N_m+1-N_on;
    Gp(2*Ap0(kp))=0;
    Gp(2*Ap0(kp)-1)=1;
    
    %K1 = 0 ; K2 = 1
    kp = N_m-N_on:-1:1;
    Gp(2*Ap0(kp))=1;
    Gp(2*Ap0(kp)-1)=0;
end
y=Gp;

== matlab function MMC_SwitchingModel_20250511/ /Sinus Modulation + Sorting Algorithm/Subsystem1/MATLAB Function1 ==
  data: ordre input; y output; sens input; N_on input
function y = fcn(ordre,sens,N_on)

N_m = length(ordre);
Gp = zeros(1,2*N_m);
Ap0=ordre;

%% Sens positif (sens = 1)
if sens==1         % ON les condensateurs les moins chargés
    
    %K1 = 1 ; K2 = 0
    kp = 1:N_on;
    Gp(2*Ap0(kp))=0;
    Gp(2*Ap0(kp)-1)=1;
    
    %K1 = 0 ; K2 = 1
    kp = N_on+1:N_m;
    Gp(2*Ap0(kp))=1;
    Gp(2*Ap0(kp)-1)=0;

else            % ON les condensateurs les plus chargés
    
    %K1 = 1 ; K2 = 0
    kp = N_m:-1:N_m+1-N_on;
    Gp(2*Ap0(kp))=0;
    Gp(2*Ap0(kp)-1)=1;
    
    %K1 = 0 ; K2 = 1
    kp = N_m-N_on:-1:1;
    Gp(2*Ap0(kp))=1;
    Gp(2*Ap0(kp)-1)=0;
end
y=Gp;

== matlab function MMC_SwitchingModel_20250511/ /Sinus Modulation + Sorting Algorithm/Number_of_Module_to_SWITCH/Number_Module_Switch_Function2 ==
  data: Nu output; P input
function Nu = fcn(P)

s=0;

for k = 1:2:length(P)
    s=s+P(k);
end

Nu=s;

== matlab function MMC_SwitchingModel_20250511/ /Sinus Modulation + Sorting Algorithm/Subsystem3/Tri phase/Tri1 ==
  data: ordre output; Vcp input; i input; sens output
function [ordre,sens] = fcn(Vcp, i)

[~, ordre] = sort(Vcp);

if i > 0 
    sens = 1;
else 
    sens = 0;
end

== matlab function MMC_SwitchingModel_20250511/ /Sinus Modulation + Sorting Algorithm/Subsystem3/Tri phase/Tri2 ==
  data: ordre output; Vcp input; i input; sens output
function [ordre,sens] = fcn(Vcp, i)

[~, ordre] = sort(Vcp);

if i > 0 
    sens = 1;
else 
    sens = 0;
end

== matlab function MMC_SwitchingModel_20250511/ /Sinus Modulation + Sorting Algorithm/Subsystem2/MATLAB Function2 ==
  data: ordre input; y output; sens input; N_on input
function y = fcn(ordre,sens,N_on)

N_m = length(ordre);
Gp = zeros(1,2*N_m);
Ap0=ordre;

%% Sens positif (sens = 1)
if sens==1         % ON les condensateurs les moins chargés
    
    %K1 = 1 ; K2 = 0
    kp = 1:N_on;
    Gp(2*Ap0(kp))=0;
    Gp(2*Ap0(kp)-1)=1;
    
    %K1 = 0 ; K2 = 1
    kp = N_on+1:N_m;
    Gp(2*Ap0(kp))=1;
    Gp(2*Ap0(kp)-1)=0;

else            % ON les condensateurs les plus chargés
    
    %K1 = 1 ; K2 = 0
    kp = N_m:-1:N_m+1-N_on;
    Gp(2*Ap0(kp))=0;
    Gp(2*Ap0(kp)-1)=1;
    
    %K1 = 0 ; K2 = 1
    kp = N_m-N_on:-1:1;
    Gp(2*Ap0(kp))=1;
    Gp(2*Ap0(kp)-1)=0;
end
y=Gp;

== matlab function MMC_SwitchingModel_20250511/ /Sinus Modulation + Sorting Algorithm/Number_of_Module_to_SWITCH/MATLAB Function4 ==
  data: Nu output; P input
function Nu = fcn(P)

s=0;

for k = 1:2:length(P)
    s=s+P(k);
end

Nu=s;

== matlab function MMC_SwitchingModel_20250511/ /Sinus Modulation + Sorting Algorithm/Number_of_Module_to_SWITCH/MATLAB Function1 ==
  data: Nu output; P input
function Nu = fcn(P)

s=0;

for k = 1:2:length(P)
    s=s+P(k);
end

Nu=s;

== matlab function MMC_SwitchingModel_20250511/ /Sinus Modulation + Sorting Algorithm/Subsystem2/Tri phase/Tri1 ==
  data: ordre output; Vcp input; i input; sens output
function [ordre,sens] = fcn(Vcp, i)

[~, ordre] = sort(Vcp);

if i > 0 
    sens = 1;
else 
    sens = 0;
end

== matlab function MMC_SwitchingModel_20250511/ /Sinus Modulation + Sorting Algorithm/Subsystem2/Tri phase/Tri2 ==
  data: ordre output; Vcp input; i input; sens output
function [ordre,sens] = fcn(Vcp, i)

[~, ordre] = sort(Vcp);

if i > 0 
    sens = 1;
else 
    sens = 0;
end
